simulink model "roboTemplate"  (Simulink 9.1)
settings: Solver=ode3  StartTime=tSim(1)  StopTime=tSim(end)  FixedStep=tStep  RelTol=1e-3  EnableMultiTasking=on
values from neighbouring files (symbols this model uses):
  A = [0 1 0 0 0 0;     9.84 -0.33 -6.9 0.08 -10.85 0;     0 0 0 1 0 0;     -115.14 -0.01 -0.28 -0.83 108.56 0;     0 0 0 0 0 1;     -770.27 1e-16 2*10^-15 -5.55 792.07 0]    [reglerInit.m]
  alpha_wMax = pi/6    (= 0.523598775598)    [roboMain.m]
  b = 0.02    [roboMain.m]
  B = [0;     -42.95;     0;     429.59;     0;     2931.20]    [reglerInit.m]
  C = [0 0 1 0 0 0;     0 0 0 0 0 1]    [reglerInit.m]
  d_w = 0.4    [roboMain.m]
  f_r = 7.2e-3    (= 0.0072)    [roboMain.m]
  g = 9.81    [roboMain.m]
  IC = [alpha_wStart alpha_w_dotStart xStart x_dotStart alpha_sStart alpha_s_dotStart]    [roboMain.m]
  J_r = 1/2*m_r*r^2    (= 4.0344e-05)    [roboMain.m]
  J_w = 1/12*m_w*(b^2+L^2)    (= 1.20033333333)    [roboMain.m]
  K_LQR = lqr(A,B,Q,R)    [reglerInit.m]
  k_w = 2    [roboMain.m]
  L = 1.2    [roboMain.m]
  L_s = 0.15    [roboMain.m]
  m_r = 0.048    [roboMain.m]
  m_s = 0.8    [roboMain.m]
  m_w = 10    [roboMain.m]
  Mmax = 0.2    [roboMain.m]
  Pmax = wMmax*Mmax    (= 3.56)    [roboMain.m]
  r = 0.041    [roboMain.m]
  Stoerung1 = .1    (= 0.1)    [roboMain.m]
  umax = 100    [roboMain.m]
  wMmax = 17.8    [roboMain.m]
libraries: simulink x1
settings Model: Creator=loehning  LastModifiedBy=AG
settings DataIOCC: SignalLoggingSaveFormat=ModelDataLogs
settings OptimizationCC: ExpressionDepthLimit=2147483647
settings DebuggingCC: SolverPrmCheckMsg=warning  FcnCallInpInsideContextMsg=warning  StateNameClashWarn=warning
settings GRTTargetCC: GeneratePreprocessorConditionals=Disable all
settings ConfigComp: CovSFcnEnable=off

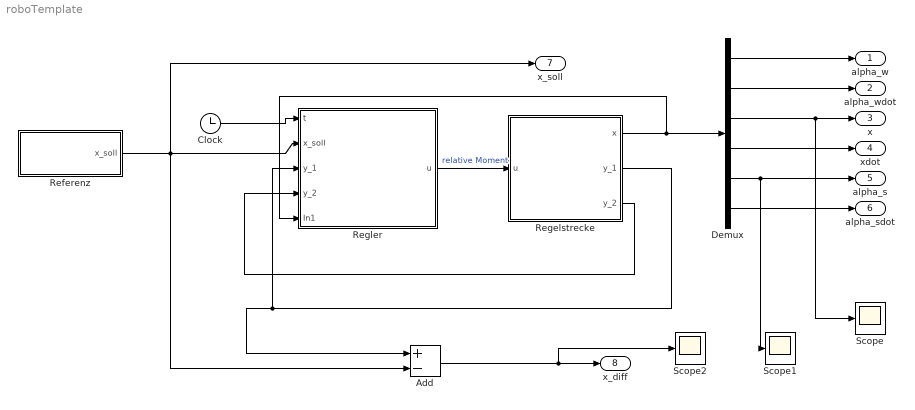
== system roboTemplate ==
  Add : Sum  Inputs=+-
  Clock : Clock
  Demux : Demux  Outputs=6
  Referenz : Subsystem
  Regelstrecke : Subsystem
  Regler : Subsystem
  Scope : Scope
  Scope1 : Scope
  Scope2 : Scope
  alpha_w : Outport
  alpha_wdot : Outport  Port=2
  x : Outport  Port=3
  xdot : Outport  Port=4
  alpha_s : Outport  Port=5
  alpha_sdot : Outport  Port=6
  x_soll : Outport  Port=7
  x_diff : Outport  Port=8
  wires:
  Regelstrecke/3(y_2) -> Regler/4(y_2)
  Regelstrecke/2(y_1) -> Add/1, Regler/3(y_1)
  Regler/1(u) -> Regelstrecke/1("u ")  "relative Moment"
  Regelstrecke/1(x) -> Regler/5(In1), Demux/1
  Clock/1 -> Regler/1(t)
  Demux/2 -> alpha_wdot/1
  Demux/6 -> alpha_sdot/1
  Demux/4 -> xdot/1
  Referenz/1("x_soll ") -> x_soll/1, Regler/2("x_soll "), Add/2
  Add/1 -> Scope2/1, x_diff/1
  Demux/5 -> Scope1/1, alpha_s/1
  Demux/3 -> Scope/1, x/1
  Demux/1 -> alpha_w/1

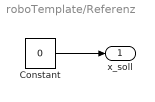
== system roboTemplate/Referenz ==
  Constant : Constant  Value=0
  "x_soll " : Outport
  wires:
  Constant/1 -> "x_soll "/1

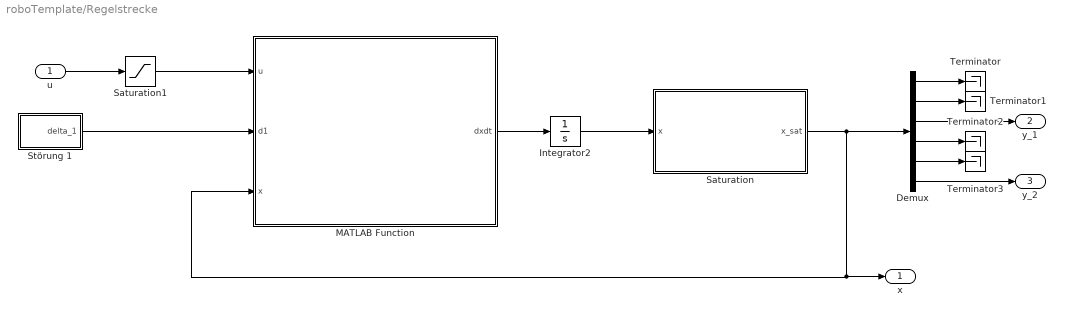
== system roboTemplate/Regelstrecke ==
  "u " : Inport
  Demux : Demux  Outputs=6
  Integrator2 : Integrator  InitialCondition=IC
  MATLAB Function : MATLAB Function  TreatAsAtomicUnit=on
  "Saturation " : MATLAB Function  TreatAsAtomicUnit=on
  Saturation1 : Saturate  UpperLimit=umax  LowerLimit=-umax
  Störung 1 : Subsystem
  Terminator{,1..3} (4 alike) : Terminator
  x : Outport
  y_1 : Outport  Port=2
  y_2 : Outport  Port=3
  wires:
  MATLAB Function/1(dxdt) -> Integrator2/1
  Störung 1/1("delta_1 ") -> MATLAB Function/2(d1)
  "Saturation "/1(x_sat) -> Demux/1, MATLAB Function/3(x), x/1
  Integrator2/1 -> "Saturation "/1(x)
  Demux/3 -> y_1/1
  Demux/6 -> y_2/1
  "u "/1 -> Saturation1/1
  Saturation1/1 -> MATLAB Function/1(u)
  Demux/1 -> Terminator/1
  Demux/2 -> Terminator1/1
  Demux/5 -> Terminator3/1
  Demux/4 -> Terminator2/1

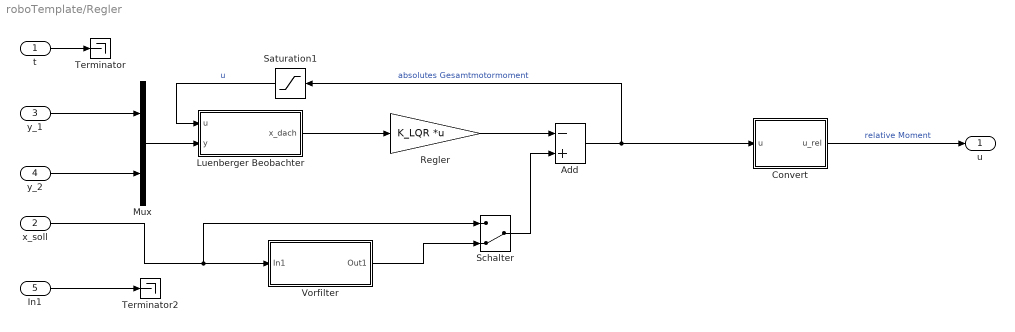
== system roboTemplate/Regler ==
  t : Inport
  "x_soll " : Inport  Port=2
  y_1 : Inport  Port=3
  y_2 : Inport  Port=4
  In1 : Inport  Port=5
  " Schalter " : ManualSwitch  CurrentSetting=0
  Add : Sum  Inputs=-+
  Convert : MATLAB Function  TreatAsAtomicUnit=on
  Luenberger Beobachter : Subsystem
  Mux : Mux  Inputs=2
  Regler : Gain  Gain=K_LQR  Multiplication=Matrix(K*u)
  Saturation1 : Saturate  UpperLimit=umax  LowerLimit=-umax
  Terminator : Terminator
  Terminator2 : Terminator
  Vorfilter : Subsystem
  u : Outport
  wires:
  t/1 -> Terminator/1
  y_1/1 -> Mux/1
  y_2/1 -> Mux/2
  Regler/1 -> Add/1
  Mux/1 -> Luenberger Beobachter/2(y)
  Saturation1/1 -> Luenberger Beobachter/1(u)  "u"
  Add/1 -> Convert/1(u), Saturation1/1  "absolutes Gesamtmotormoment"
  "x_soll "/1 -> " Schalter "/1, Vorfilter/1(In1)
  Luenberger Beobachter/1(x_dach) -> Regler/1
  Convert/1(u_rel) -> u/1  "relative Moment"
  In1/1 -> Terminator2/1
  Vorfilter/1(Out1) -> " Schalter "/2
  " Schalter "/1 -> Add/2

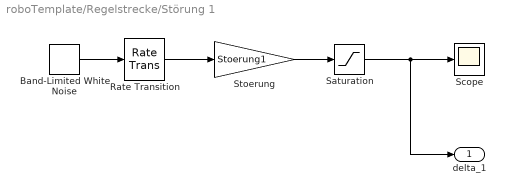
== system roboTemplate/Regelstrecke/Störung 1 ==
  Band-Limited White Noise : simulink/Sources/Band-Limited White Noise  Cov=stoerungNoisePower  Ts=0.025  seed=stoerungSeed_1
  Rate Transition : RateTransition
  Saturation : Saturate  UpperLimit=3  LowerLimit=-3
  Scope : Scope
  Stoerung : Gain  Gain=Stoerung1
  "delta_1 " : Outport
  wires:
  Band-Limited White Noise/1 -> Rate Transition/1
  Rate Transition/1 -> Stoerung/1
  Stoerung/1 -> Saturation/1
  Saturation/1 -> "delta_1 "/1, Scope/1

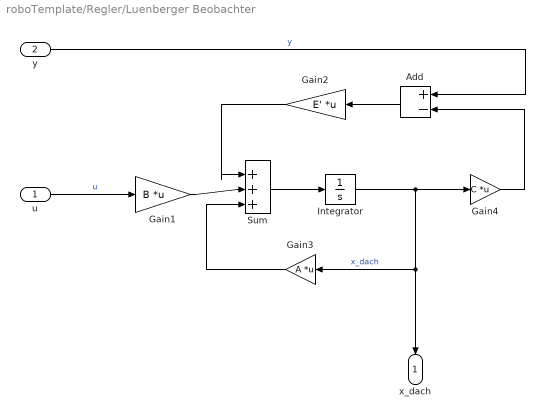
== system roboTemplate/Regler/Luenberger Beobachter ==
  u : Inport
  y : Inport  Port=2
  Add : Sum  Inputs=+-
  Gain1 : Gain  Gain=B  Multiplication=Matrix(K*u)
  Gain2 : Gain  Gain=E'  Multiplication=Matrix(K*u)
  Gain3 : Gain  Gain=A  Multiplication=Matrix(K*u)
  Gain4 : Gain  Gain=C  Multiplication=Matrix(K*u)
  Integrator : Integrator  InitialCondition=IC
  Sum : Sum  Inputs=|+++
  x_dach : Outport
  wires:
  Integrator/1 -> Gain3/1, x_dach/1, Gain4/1  "x_dach"
  Gain3/1 -> Sum/3
  Gain2/1 -> Sum/1
  Add/1 -> Gain2/1
  Gain1/1 -> Sum/2
  Gain4/1 -> Add/2
  Sum/1 -> Integrator/1
  u/1 -> Gain1/1  "u"
  y/1 -> Add/1  "y"

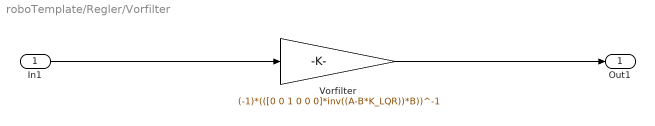
== system roboTemplate/Regler/Vorfilter ==
  In1 : Inport
  Vorfilter : Gain  Gain=(-1)*(([0 0 1 0 0 0]*inv((A-B*K_LQR))*B))^-1
  Out1 : Outport
  wires:
  In1/1 -> Vorfilter/1
  Vorfilter/1 -> Out1/1

== matlab function Regelstrecke/MATLAB Function ==
  data: u input double; d1 input double; dxdt output double size=[1 6]; x input double size=[1 6]; g parameter double; m_w parameter double; k_w parameter double; d_w parameter double; L parameter double; b parameter double; J_w parameter double; L_s parameter double; m_s parameter double; Mmax parameter double; wMmax parameter double; Pmax parameter double; umax parameter double; m_r parameter double; f_r parameter double; J_r parameter double; r parameter double
function dxdt   = dynamikStrecke(u, d1, x, g, m_w, k_w, d_w, L, b, J_w, L_s, m_s, Mmax, wMmax, Pmax, umax, m_r, f_r, J_r, r)
% Dynamik von Wippe und Segway

%Motormoment
P = (u+d1)/umax*Pmax; %Leistung eines Motors
M_max = sqrt(abs(P))/9.434;
M = 2*sign(u)*M_max; % Gesamtmoment
%M=u;
%Reibung
F_r = f_r*x(4)*g*(m_r+m_s)*cos(x(1));

%Massenmatrix
d_alpha = x(5)-x(1);
MM = [J_w+m_r*(x(3)^2+3/2*r^2)+m_s*(r^2+x(3)^2) -((3/2*m_r+m_s)*r+m_s*L_s*cos(d_alpha)) m_s*L_s*(r*cos(d_alpha)-x(3)*sin(d_alpha));
     -(3/2*m_r+m_s)*r 3/2*m_r+m_s -m_s*L_s*cos(d_alpha);
     m_s*L_s*(r*cos(d_alpha)-x(3)*sin(d_alpha)) -m_s*L_s*cos(d_alpha) m_s*L_s^2]; 

% Bewegungsgleichungen 
dxdt = zeros(1,6);  
dxdt(1)=x(2); %alpha_w
dxdt(3)=x(4); %x
dxdt(5)= x(6); %alpha_s

acc = MM^-1*[-(2*(m_r+m_s)*x(3)-m_s*L_s*sin(d_alpha))*x(4)*x(2)-m_s*L_s*sin(d_alpha)*x(4)*x(6)+m_s*L_s*x(6)^2*(r*sin(d_alpha)+x(3)*cos(d_alpha))-k_w*x(1)-(m_r+m_s)*g*(x(3)*cos(x(1))-r*sin(x(1)))-M-d_w*x(2);
                                    -m_s*L_s*sin(d_alpha)*x(6)^2+(m_r+m_s)*x(3)*x(2)^2-(m_r+m_s)*g*sin(x(1))+1/r*M-F_r;
                                   -(r*sin(d_alpha)+x(3)*cos(d_alpha))*x(2)^2*m_s*L_s+g*m_s*L_s*sin(x(5))+M ];               % alpha_w_dot, x_dot, alpha_s_dot 

dxdt(2) = acc(1);
dxdt(4) = acc(2);
dxdt(6) = acc(3);

== matlab function Regler/Convert ==
  data: u input double; u_rel output double
function u_rel = fcn(u)    % u : u_Schlange: absolute u bzw. 
Pmax = 3.56;

u_rel = 9.434^2/4*u^2*sign(u/2)*100/Pmax;

== matlab function Regelstrecke/Saturation  ==
  data: x input double; alpha_wMax parameter double; x_sat output double; L parameter double
function x_sat  = fcn(x, alpha_wMax,  L)


x_sat = x;

%Saturation in alpha_w und alpha_w_dot
if x(1) >= alpha_wMax
    x_sat(1) = alpha_wMax;
    if x(2) > 0
        x_sat(2) = 0;
    end
end

if x(1) <= -alpha_wMax
    x_sat(1) = -alpha_wMax;
    if x(2) < 0
        x_sat(2) = 0;
    end
end

%Saturation in x
if x(3) >= L/2
    x_sat(3) = L/2;
    x_sat(4) = 0; %Roboter fällt herunter!!!!
end

if x(3) <= -L/2
    x_sat(3) = -L/2;
    x_sat(4) = 0; %Roboter fällt herunter!!!!
end

%Saturation in alpha_s
delta_alpha = x(5)-x(1);
if delta_alpha >= pi/2
    x_sat(5) = pi/2+x(1);
    x_sat(6) = x_sat(2); %Roboter ist umgekippt!!!!
end

if delta_alpha <= -pi/2
    x_sat(5) = -pi/2+x(1);
    x_sat(6) = x_sat(2); %Roboter ist umgekippt!!!!
end
